simulink model "WFXXPIDa"  (Simulink 8.3)
settings: Solver=ode5  SolverMode=SingleTasking  StartTime=0.0  StopTime=8000  FixedStep=5  RelTol=1e-3
settings Model: Creator=Zhu Supeng  LastModifiedBy=Zhu Supeng
settings DataIOCC: SignalLoggingName=sigsOut
settings DebuggingCC: SaveWithParameterizedLinksMsg=none  SignalResolutionControl=TryResolveAllWithWarning  SolverPrmCheckMsg=none  MultiTaskDSMMsg=warning  MultiTaskCondExecSysMsg=none  StateNameClashWarn=none
settings HardwareCC: TargetUnknown=on
settings RTWCC: IncludeERTFirstTime=on

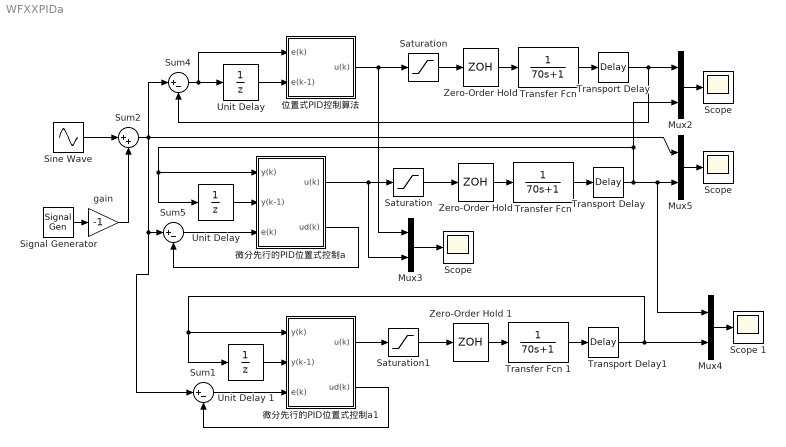
== system WFXXPIDa ==
  " Scope" : Scope
      settings: YMin=-1.5  YMax=1.5  SaveName=WFXXPIDau  MaxDataPoints=500000
  Mux{2..5} (4 alike) : Mux  Inputs=2
  Saturation : Saturate  UpperLimit=10  LowerLimit=-10
  "Saturation " : Saturate  UpperLimit=10  LowerLimit=-10
  Saturation1 : Saturate  UpperLimit=10  LowerLimit=-10
  Scope : Scope
      settings: YMin=-1.5  YMax=1.5  SaveName=WFXXPIDPIDay  MaxDataPoints=500000
  "Scope " : Scope
      settings: TimeRange=3200  YMin=-0.402515  YMax=0.797485  SaveName=WFXXPIDary  MaxDataPoints=500000
  Scope 1 : Scope
      settings: TimeRange=3200  YMin=-0.402515  YMax=0.797485  SaveName=WFXXPIDary1  MaxDataPoints=500000
  Signal Generator : SignalGenerator  WaveForm=square  Frequency=0.0005*pi  Units=rad/sec
  Sine Wave : Sin  Amplitude=0.05  Frequency=0.03*pi  SampleTime=0
  Sum1 : Sum  Inputs=|+-  SaturateOnIntegerOverflow=on
  Sum2 : Sum  Inputs=|++  SaturateOnIntegerOverflow=on
  Sum4 : Sum  Inputs=|+-  SaturateOnIntegerOverflow=on
  Sum5 : Sum  Inputs=|+-  SaturateOnIntegerOverflow=on
  Transfer Fcn : TransferFcn  Denominator=[70 1]
  "Transfer Fcn " : TransferFcn  Denominator=[70 1]
  Transfer Fcn 1 : TransferFcn  Denominator=[70 1]
  Transport Delay : TransportDelay  DelayTime=80
  "Transport Delay " : TransportDelay  DelayTime=80
  Transport Delay1 : TransportDelay  DelayTime=80
  Unit Delay : UnitDelay  SampleTime=20
  "Unit Delay " : UnitDelay  SampleTime=20
  Unit Delay 1 : UnitDelay  SampleTime=20
  Zero-Order Hold : ZeroOrderHold  SampleTime=20
  "Zero-Order Hold " : ZeroOrderHold  SampleTime=20
  Zero-Order Hold 1 : ZeroOrderHold  SampleTime=20
  gain : Gain  Gain=-1  SaturateOnIntegerOverflow=on  OutDataTypeStr=Inherit: Same as input  ParamDataTypeStr=Inherit: Same as input
  "位置式PID控制算法 " : Subsystem
  微分先行的PID位置式控制a : Subsystem
  微分先行的PID位置式控制a1 : Subsystem
  wires:
  "Transfer Fcn "/1 -> Transport Delay/1
  微分先行的PID位置式控制a/1(u(k)) -> Saturation/1, Mux3/2
  "Zero-Order Hold "/1 -> "Transfer Fcn "/1
  Mux5/1 -> "Scope "/1
  Transport Delay/1 -> Mux4/1, Mux5/2, 微分先行的PID位置式控制a/1(y(k)), "Unit Delay "/1, Mux2/2
  Sum5/1 -> 微分先行的PID位置式控制a/3(e(k))
  Transfer Fcn/1 -> "Transport Delay "/1
  "位置式PID控制算法 "/1(u(k)) -> "Saturation "/1, Mux3/1
  Sum4/1 -> Unit Delay/1, "位置式PID控制算法 "/1(e(k))
  Zero-Order Hold/1 -> Transfer Fcn/1
  Mux2/1 -> Scope/1
  "Transport Delay "/1 -> Mux2/1, Sum4/2
  Unit Delay/1 -> "位置式PID控制算法 "/2(e(k-1))
  "Unit Delay "/1 -> 微分先行的PID位置式控制a/2(y(k-1))
  Sine Wave/1 -> Sum2/1
  Signal Generator/1 -> gain/1
  gain/1 -> Sum2/2
  微分先行的PID位置式控制a/2(ud(k)) -> Sum5/2
  Saturation/1 -> "Zero-Order Hold "/1
  "Saturation "/1 -> Zero-Order Hold/1
  Mux3/1 -> " Scope"/1
  Sum2/1 -> Sum4/1, Sum1/1, Sum5/1, Mux5/1
  Transfer Fcn 1/1 -> Transport Delay1/1
  微分先行的PID位置式控制a1/1(u(k)) -> Saturation1/1
  Zero-Order Hold 1/1 -> Transfer Fcn 1/1
  Mux4/1 -> Scope 1/1
  Sum1/1 -> 微分先行的PID位置式控制a1/3(e(k))
  Unit Delay 1/1 -> 微分先行的PID位置式控制a1/2(y(k-1))
  微分先行的PID位置式控制a1/2(ud(k)) -> Sum1/2
  Saturation1/1 -> Zero-Order Hold 1/1
  Transport Delay1/1 -> Unit Delay 1/1, 微分先行的PID位置式控制a1/1(y(k)), Mux4/2

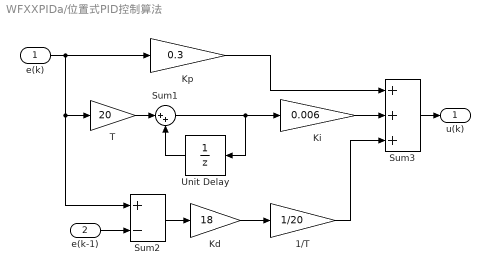
== system WFXXPIDa/位置式PID控制算法  ==
  e(k) : Inport
  e(k-1) : Inport  Port=2
  1/T : Gain  Gain=1/20  SaturateOnIntegerOverflow=on  OutDataTypeStr=Inherit: Same as input  ParamDataTypeStr=Inherit: Same as input
  Kd : Gain  Gain=18  SaturateOnIntegerOverflow=on  OutDataTypeStr=Inherit: Same as input  ParamDataTypeStr=Inherit: Same as input
  Ki : Gain  Gain=0.006  SaturateOnIntegerOverflow=on  OutDataTypeStr=Inherit: Same as input  ParamDataTypeStr=Inherit: Same as input
  Kp : Gain  Gain=0.3  SaturateOnIntegerOverflow=on  OutDataTypeStr=Inherit: Same as input  ParamDataTypeStr=Inherit: Same as input
  Sum1 : Sum  Inputs=|++  SaturateOnIntegerOverflow=on
  Sum2 : Sum  Inputs=+-  SaturateOnIntegerOverflow=on
  Sum3 : Sum  Inputs=+++  SaturateOnIntegerOverflow=on
  T : Gain  Gain=20  SaturateOnIntegerOverflow=on  OutDataTypeStr=Inherit: Same as input  ParamDataTypeStr=Inherit: Same as input
  Unit Delay : UnitDelay  SampleTime=20
  u(k) : Outport
  wires:
  Sum2/1 -> Kd/1
  e(k)/1 -> Kp/1, Sum2/1, T/1
  Kp/1 -> Sum3/1
  Ki/1 -> Sum3/2
  Sum3/1 -> u(k)/1
  Kd/1 -> 1/T/1
  e(k-1)/1 -> Sum2/2
  1/T/1 -> Sum3/3
  Sum1/1 -> Unit Delay/1, Ki/1
  Unit Delay/1 -> Sum1/2
  T/1 -> Sum1/1

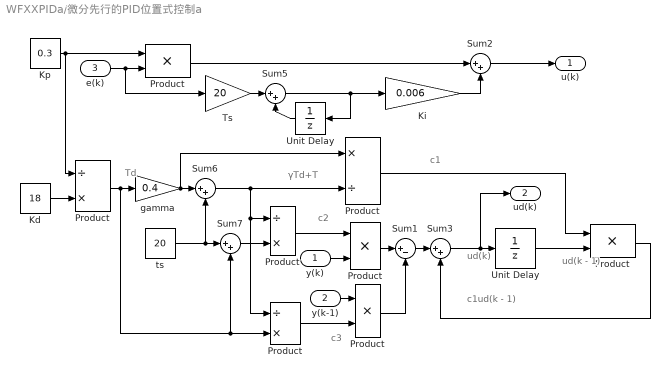
== system WFXXPIDa/微分先行的PID位置式控制a ==
  note: c1ud(k－1)
  note: c2
  note: c3
  note: c1
  note: ud(k－1)
  note: ud(k)
  note: Td
  note: γTd+T
  y(k) : Inport
  y(k-1) : Inport  Port=2
  e(k) : Inport  Port=3
  "  Product " : Product  SaturateOnIntegerOverflow=on  OutDataTypeStr=Inherit: Same as first input
  "  Product  " : Product  Inputs=/*  SaturateOnIntegerOverflow=on  OutDataTypeStr=Inherit: Same as first input
  "  Product   " : Product  SaturateOnIntegerOverflow=on  OutDataTypeStr=Inherit: Same as first input
  " Product" : Product  Inputs=*/  SaturateOnIntegerOverflow=on  OutDataTypeStr=Inherit: Same as first input
  " Product " : Product  Inputs=/*  SaturateOnIntegerOverflow=on  OutDataTypeStr=Inherit: Same as first input
  " Product  " : Product  SaturateOnIntegerOverflow=on  OutDataTypeStr=Inherit: Same as first input
  " Product   " : Product  Inputs=/*  SaturateOnIntegerOverflow=on  OutDataTypeStr=Inherit: Same as first input
  " Unit Delay " : UnitDelay  SampleTime=20
  Kd : Constant  Value=18
  Ki : Gain  Gain=0.006  SaturateOnIntegerOverflow=on  OutDataTypeStr=Inherit: Same as input  ParamDataTypeStr=Inherit: Same as input
  Kp : Constant  Value=0.3
  Product : Product  SaturateOnIntegerOverflow=on  OutDataTypeStr=Inherit: Same as first input
  Sum1 : Sum  Inputs=|+-  SaturateOnIntegerOverflow=on
  Sum{2..3,5..7} (5 alike) : Sum  Inputs=|++  SaturateOnIntegerOverflow=on
  Ts : Gain  Gain=20  SaturateOnIntegerOverflow=on  OutDataTypeStr=Inherit: Same as input  ParamDataTypeStr=Inherit: Same as input
  "Unit Delay " : UnitDelay  SampleTime=20
  gamma : Gain  Gain=0.4  SaturateOnIntegerOverflow=on  OutDataTypeStr=Inherit: Same as input  ParamDataTypeStr=Inherit: Same as input
  ts : Constant  Value=20
  u(k) : Outport
  ud(k) : Outport  Port=2
  wires:
  e(k)/1 -> Ts/1, Product/2
  Ts/1 -> Sum5/1
  Sum5/1 -> "Unit Delay "/1, Ki/1
  "Unit Delay "/1 -> Sum5/2
  Product/1 -> Sum2/1
  Ki/1 -> Sum2/2
  Sum1/1 -> Sum3/1
  Sum2/1 -> u(k)/1
  Sum3/1 -> " Unit Delay "/1, ud(k)/1
  Kp/1 -> Product/1, " Product "/1
  Kd/1 -> " Product "/2
  gamma/1 -> Sum6/1, " Product"/1
  ts/1 -> Sum6/2, Sum7/1
  Sum6/1 -> " Product"/2, " Product   "/1, "  Product  "/1
  " Product "/1 -> Sum7/2, "  Product  "/2, gamma/1
  Sum7/1 -> " Product   "/2
  " Product   "/1 -> "  Product   "/1
  "  Product  "/1 -> "  Product "/2
  y(k)/1 -> "  Product   "/2
  "  Product   "/1 -> Sum1/1
  y(k-1)/1 -> "  Product "/1
  "  Product "/1 -> Sum1/2
  " Product"/1 -> " Product  "/1
  " Product  "/1 -> Sum3/2
  " Unit Delay "/1 -> " Product  "/2

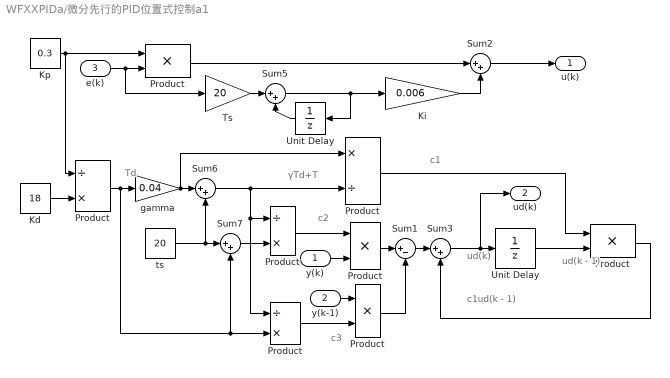
== system WFXXPIDa/微分先行的PID位置式控制a1 ==
  note: γTd+T
  note: Td
  note: ud(k)
  note: ud(k－1)
  note: c1
  note: c3
  note: c2
  note: c1ud(k－1)
  y(k) : Inport
  y(k-1) : Inport  Port=2
  e(k) : Inport  Port=3
  "  Product " : Product  SaturateOnIntegerOverflow=on  OutDataTypeStr=Inherit: Same as first input
  "  Product  " : Product  Inputs=/*  SaturateOnIntegerOverflow=on  OutDataTypeStr=Inherit: Same as first input
  "  Product   " : Product  SaturateOnIntegerOverflow=on  OutDataTypeStr=Inherit: Same as first input
  " Product" : Product  Inputs=*/  SaturateOnIntegerOverflow=on  OutDataTypeStr=Inherit: Same as first input
  " Product " : Product  Inputs=/*  SaturateOnIntegerOverflow=on  OutDataTypeStr=Inherit: Same as first input
  " Product  " : Product  SaturateOnIntegerOverflow=on  OutDataTypeStr=Inherit: Same as first input
  " Product   " : Product  Inputs=/*  SaturateOnIntegerOverflow=on  OutDataTypeStr=Inherit: Same as first input
  " Unit Delay " : UnitDelay  SampleTime=20
  Kd : Constant  Value=18
  Ki : Gain  Gain=0.006  SaturateOnIntegerOverflow=on  OutDataTypeStr=Inherit: Same as input  ParamDataTypeStr=Inherit: Same as input
  Kp : Constant  Value=0.3
  Product : Product  SaturateOnIntegerOverflow=on  OutDataTypeStr=Inherit: Same as first input
  Sum1 : Sum  Inputs=|+-  SaturateOnIntegerOverflow=on
  Sum{2..3,5..7} (5 alike) : Sum  Inputs=|++  SaturateOnIntegerOverflow=on
  Ts : Gain  Gain=20  SaturateOnIntegerOverflow=on  OutDataTypeStr=Inherit: Same as input  ParamDataTypeStr=Inherit: Same as input
  "Unit Delay " : UnitDelay  SampleTime=20
  gamma : Gain  Gain=0.04  SaturateOnIntegerOverflow=on  OutDataTypeStr=Inherit: Same as input  ParamDataTypeStr=Inherit: Same as input
  ts : Constant  Value=20
  u(k) : Outport
  ud(k) : Outport  Port=2
  wires:
  " Unit Delay "/1 -> " Product  "/2
  " Product  "/1 -> Sum3/2
  " Product"/1 -> " Product  "/1
  "  Product "/1 -> Sum1/2
  y(k-1)/1 -> "  Product "/1
  "  Product   "/1 -> Sum1/1
  y(k)/1 -> "  Product   "/2
  "  Product  "/1 -> "  Product "/2
  " Product   "/1 -> "  Product   "/1
  Sum7/1 -> " Product   "/2
  " Product "/1 -> gamma/1, "  Product  "/2, Sum7/2
  Sum6/1 -> "  Product  "/1, " Product   "/1, " Product"/2
  ts/1 -> Sum7/1, Sum6/2
  gamma/1 -> " Product"/1, Sum6/1
  Kd/1 -> " Product "/2
  Kp/1 -> " Product "/1, Product/1
  Sum3/1 -> ud(k)/1, " Unit Delay "/1
  Sum2/1 -> u(k)/1
  Sum1/1 -> Sum3/1
  Ki/1 -> Sum2/2
  Product/1 -> Sum2/1
  "Unit Delay "/1 -> Sum5/2
  Sum5/1 -> Ki/1, "Unit Delay "/1
  Ts/1 -> Sum5/1
  e(k)/1 -> Product/2, Ts/1
